simulink model "RMSimModel"  (R2023a)
settings: Solver=VariableStepAuto  StartTime=0.0  StopTime=60.0  RelTol=1e-3
model workspace (MAT data in the model file):
  A = 1
  ADownforce = 1.5
  AirDensity = 1
  Cd = 1.5
  CdDownforce = 1.4
  Crr = 0.0015
  Gravity = 9.81
  Incline = 0
  K_c = 0.2
  K_i = 0.005
  K_w = 0.0005
  MaxRPM = 2000
  TireRadius = 0.2032
  Torque = 230
  massCar = 130
  massDriver = 60
libraries: LinkedSubsytems x5
settings Model: Creator=Tre'Vaughn  LastModifiedBy=Tre'Vaughn

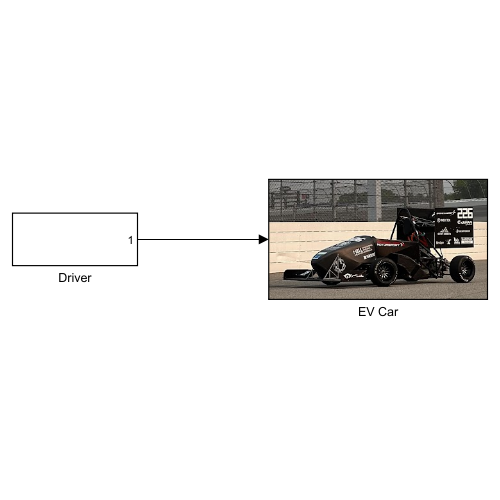
[thumbnail: Simulink's stored preview of the top-level diagram]
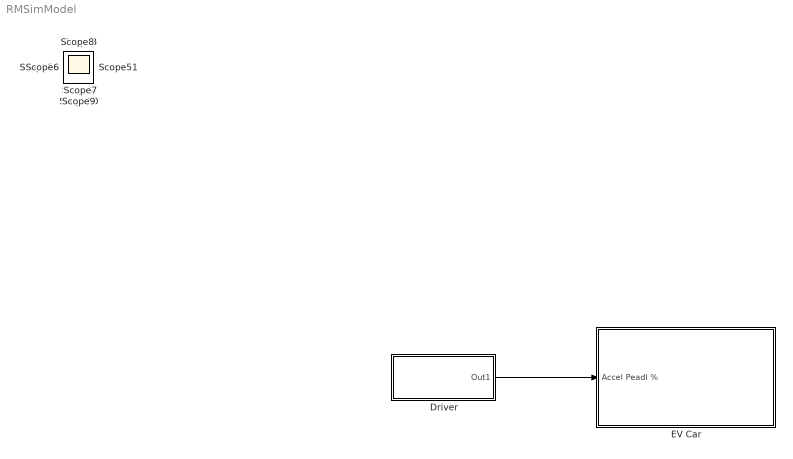
== system RMSimModel ==
  Driver : Subsystem
  EV Car : Subsystem
      mask Display: image('$imagefile'); % Use "Edit Image" on toolstrip to change.
  Scope{,1..12} (13 alike) : Scope
  wires:
  Driver/1(Out1) -> EV Car/1(Accel Peadl %)

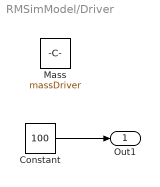
== system RMSimModel/Driver ==
  Constant : Constant  Value=100
  Mass : Constant  Value=massDriver
  Out1 : Outport
  wires:
  Constant/1 -> Out1/1

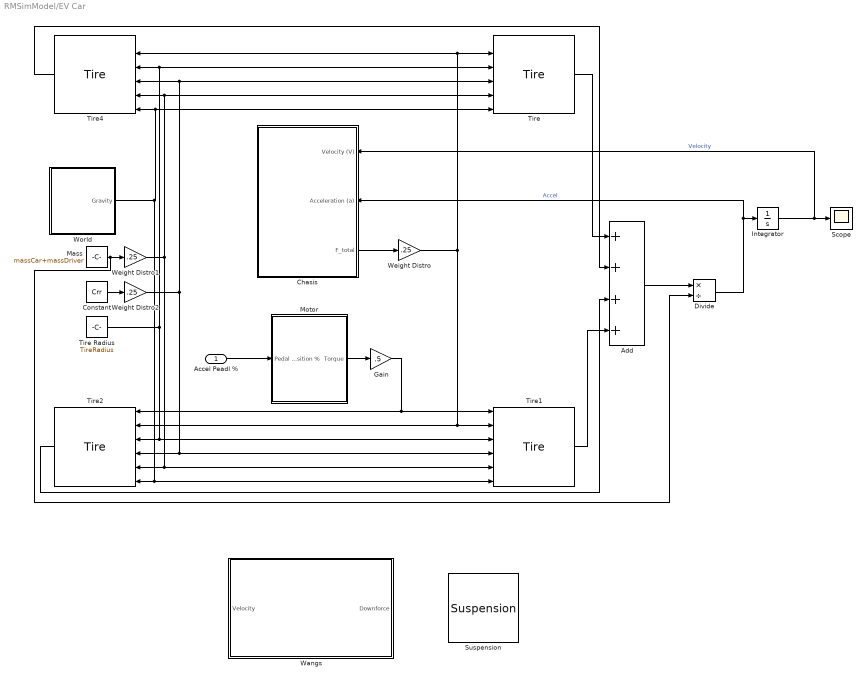
== system RMSimModel/EV Car ==
  Accel Peadl % : Inport
  Add : Sum  Inputs=++++
  Chasis : Subsystem
      settings: PortSchema="{\"entries\":[{\"content\":{\"sides\":[{\"content\":{},\"type\":\"ConnectorPlacement.EquallySpacedRectSide\",\"uuid\":\"3bf05a28-119f-4ffa-933d-d1f1ff116959\"},{\"content\":{\"connectorIds\":[\"In1\",\"In2\",\"Out1\"],\"side\":\"RIGHT\"},\"type\":\"ConnectorPlacement.EquallySpacedRectSide\",\"uuid\":\"eb63bc44-58b6-4772-bae2-bbb2fef2688c\"},{\"content\":{\"side\":\"TOP\"},\"type\":\"ConnectorPlacement.EquallySpacedRectSide\",\"uuid\":\"2e4910ff-b3b7-4eae-a46e-a8fd4b8b6d71\"},{\"content\":{\"side\":\"BOTTOM\"},\"type\":\"ConnectorPlacement.EquallySpacedRectSide\",\"uuid\":\"c70a882d-c287-4241-9fb9-cc60e98faa0b\"}]},\"type\":\"ConnectorPlacement.EquallySpacedConnector\",\"uuid\":\"e510c1be-65df-4579-86ba-56f04766634d\"}],\"packageUris\":[\"http://schema.mathworks.com/mf0/Connector/R2020b\"],\"version\":\"1.0\"}"
      mask Display: image('$imagefile'); % Use "Edit Image" on toolstrip to change.
  Constant : Constant  Value=Crr
  Divide : Product  Inputs=*/
  Gain : Gain  Gain=.5
  Integrator : Integrator
  Mass : Constant  Value=massCar+massDriver
  Motor : Subsystem
      mask Display: image('C:\Users\Tre''Vaughn\Documents\MATLAB\RMSimModel\Subsystem Pics\Motor.png'); % Use "Edit Image" on toolstrip to change.
  Scope : Scope
  Suspension : LinkedSubsytems/Suspension  SystemSampleTime=-1  VariantActivationTime=update diagram  Latency=0  AutoFrameSizeCalculation=off
  Tire{,1..2,4} (4 alike) : LinkedSubsytems/Tire  SystemSampleTime=-1  VariantActivationTime=update diagram  Latency=0  AutoFrameSizeCalculation=off
  Tire Radius : Constant  Value=TireRadius
  Wangs : Subsystem
      mask Display: image('C:\Users\Tre''Vaughn\Documents\MATLAB\RMSimModel\Subsystem Pics\Rear Wang.png'); % Use "Edit Image" on toolstrip to change.
  Weight Distro : Gain  Gain=.25
  Weight Distro1 : Gain  Gain=.25
  Weight Distro2 : Gain  Gain=.25
  World : Subsystem
      mask Display: image('C:\Users\Tre''Vaughn\Documents\MATLAB\RMSimModel\Subsystem Pics\World.png'); % Use "Edit Image" on toolstrip to change.
  wires:
  Accel Peadl %/1 -> Motor/1(Pedal Position %)
  Chasis/1(F_total) -> Weight Distro/1
  Motor/1(Torque) -> Gain/1
  Add/1 -> Divide/1
  Divide/1 -> Chasis/2(Acceleration (a)), Integrator/1  "Accel"
  Integrator/1 -> Chasis/1(Velocity (V)), Scope/1  "Velocity"
  Tire1/1 -> Add/4
  Tire/1 -> Add/1
  Tire4/1 -> Add/2
  Tire2/1 -> Add/3
  Gain/1 -> Tire2/1, Tire1/1
  World/1(Gravity) -> Tire1/6, Tire2/6, Tire4/6, Tire/6
  Tire Radius/1 -> Tire/3, Tire4/3, Tire1/3, Tire2/3
  Constant/1 -> Weight Distro2/1
  Weight Distro/1 -> Tire/2, Tire4/2, Tire2/2, Tire1/2
  Weight Distro1/1 -> Tire1/5, Tire2/5, Tire/5, Tire4/5
  Weight Distro2/1 -> Tire2/4, Tire1/4, Tire/4, Tire4/4
  Mass/1 -> Weight Distro1/1, Divide/2

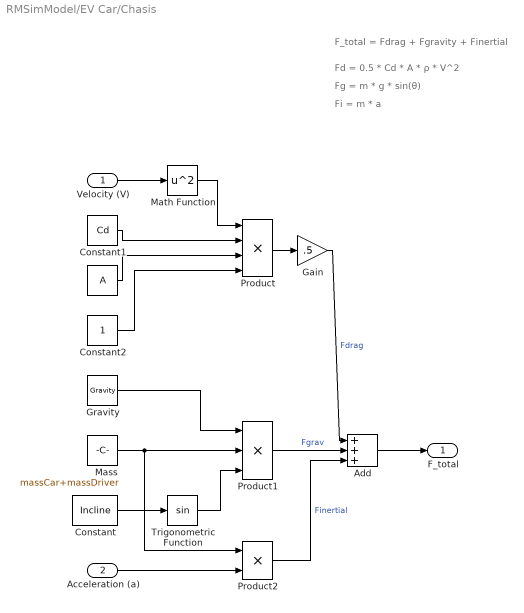
== system RMSimModel/EV Car/Chasis ==
  note: Fi = m * a
  note: Fg = m * g * sin(θ)
  note: Fd = 0.5 * Cd * A * ρ * V^2
  note: F_total = Fdrag + Fgravity + Finertial
  Velocity (V) : Inport
  Acceleration (a) : Inport  Port=2
  " " : Constant  Value=A
  Add : Sum  Inputs=+++
  Constant : Constant  Value=Incline
  Constant1 : Constant  Value=Cd
  Constant2 : Constant
  Gain : Gain  Gain=.5
  Gravity : Constant  Value=Gravity
  Mass : Constant  Value=massCar+massDriver
  Math Function : Math  Operator=square
  Product : Product  Inputs=4
  Product1 : Product  Inputs=3
  Product2 : Product
  Trigonometric Function : Trigonometry
  F_total : Outport
  wires:
  Gain/1 -> Add/1  "Fdrag"
  Velocity (V)/1 -> Math Function/1
  Product/1 -> Gain/1
  Math Function/1 -> Product/1
  Constant1/1 -> Product/2
  " "/1 -> Product/3
  Constant2/1 -> Product/4
  Constant/1 -> Trigonometric Function/1
  Mass/1 -> Product2/1, Product1/2
  Gravity/1 -> Product1/1
  Trigonometric Function/1 -> Product1/3
  Product1/1 -> Add/2  "Fgrav"
  Acceleration (a)/1 -> Product2/2
  Product2/1 -> Add/3  "Finertial"
  Add/1 -> F_total/1

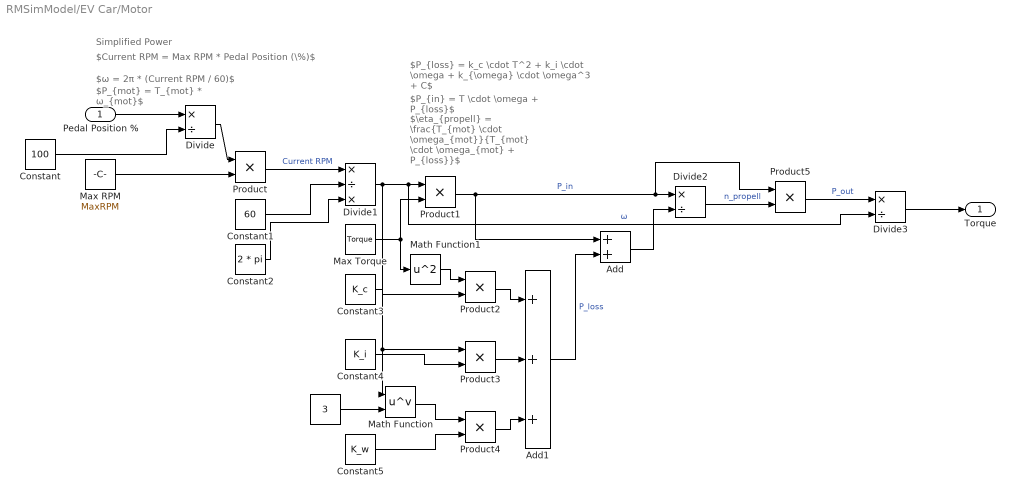
== system RMSimModel/EV Car/Motor ==
  note: Simplified Power
  note: $ω = 2π * (Current RPM / 60)$
  note: $Current RPM = Max RPM * Pedal Position (\%)$
  note: $\eta_{propell} = \frac{T_{mot} \cdot \omega_{mot}}{T_{mot} \cdot \omega_{mot} + P_{loss}}$
  note: $P_{in} = T \cdot \omega + P_{loss}$
  note: $P_{loss} = k_c \cdot T^2 + k_i \cdot \omega + k_{\omega} \cdot \omega^3 + C$
  note: $P_{mot} = T_{mot} * ω_{mot}$
  Pedal Position % : Inport
  " " : Constant  Value=3
  Add : Sum
  Add1 : Sum  Inputs=+++
  Constant : Constant  Value=100
  Constant1 : Constant  Value=60
  Constant2 : Constant  Value=2 * pi
  Constant3 : Constant  Value=K_c
  Constant4 : Constant  Value=K_i
  Constant5 : Constant  Value=K_w
  Divide : Product  Inputs=*/
  Divide1 : Product  Inputs=*/*
  Divide2 : Product  Inputs=*/
  Divide3 : Product  Inputs=*/
  Math Function : Math  Operator=pow
  Math Function1 : Math  Operator=square
  Max RPM : Constant  Value=MaxRPM
  Max Torque : Constant  Value=Torque
  Product{,1..5} (6 alike) : Product
  Torque : Outport
  wires:
  Pedal Position %/1 -> Divide/1
  Max RPM/1 -> Product/2
  Product/1 -> Divide1/1  "Current RPM"
  Constant/1 -> Divide/2
  Divide/1 -> Product/1
  Constant1/1 -> Divide1/2
  Constant2/1 -> Divide1/3
  Divide1/1 -> Math Function/1, Product3/1, Divide3/2, Product1/1  "ω"
  Max Torque/1 -> Product1/2, Math Function1/1
  Product1/1 -> Add/1, Product5/1, Divide2/1  "P_in"
  Add/1 -> Divide2/2
  Constant3/1 -> Product2/2
  Constant4/1 -> Product3/2
  " "/1 -> Math Function/2
  Math Function/1 -> Product4/1
  Constant5/1 -> Product4/2
  Math Function1/1 -> Product2/1
  Product3/1 -> Add1/2
  Product2/1 -> Add1/1
  Product4/1 -> Add1/3
  Add1/1 -> Add/2  "P_loss"
  Divide2/1 -> Product5/2  "n_propell"
  Product5/1 -> Divide3/1  "P_out"
  Divide3/1 -> Torque/1

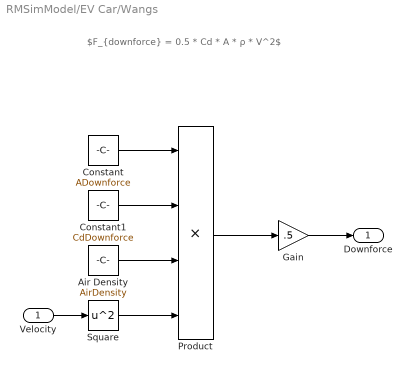
== system RMSimModel/EV Car/Wangs ==
  note: $F_{downforce} = 0.5 * Cd * A * ρ * V^2$
  Velocity : Inport
  Air Density : Constant  Value=AirDensity
  Constant : Constant  Value=ADownforce
  Constant1 : Constant  Value=CdDownforce
  Gain : Gain  Gain=.5
  Product : Product  Inputs=4
  Square : Math  Operator=square
  Downforce : Outport
  wires:
  Gain/1 -> Downforce/1
  Constant1/1 -> Product/2
  Product/1 -> Gain/1
  Air Density/1 -> Product/3
  Velocity/1 -> Square/1
  Constant/1 -> Product/1
  Square/1 -> Product/4

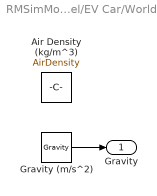
== system RMSimModel/EV Car/World ==
  Air Density (kg/m^3) : Constant  Value=AirDensity
  Gravity (m/s^2) : Constant  Value=Gravity
  Gravity : Outport
  wires:
  Gravity (m/s^2)/1 -> Gravity/1
